simulink model "monosim"  (Simulink 7.7)
settings: Solver=ode45  StartTime=0.0  StopTime=10.0  MaxStep=0.01  RelTol=1e-3
values from neighbouring files (symbols this model uses):
  beta = 0.001    [teste.m]
undefined symbols (not defined in the file or in its folder): J, K, T
settings Model: Creator=ClaudiaPinto  LastModifiedBy=ClaudiaPinto

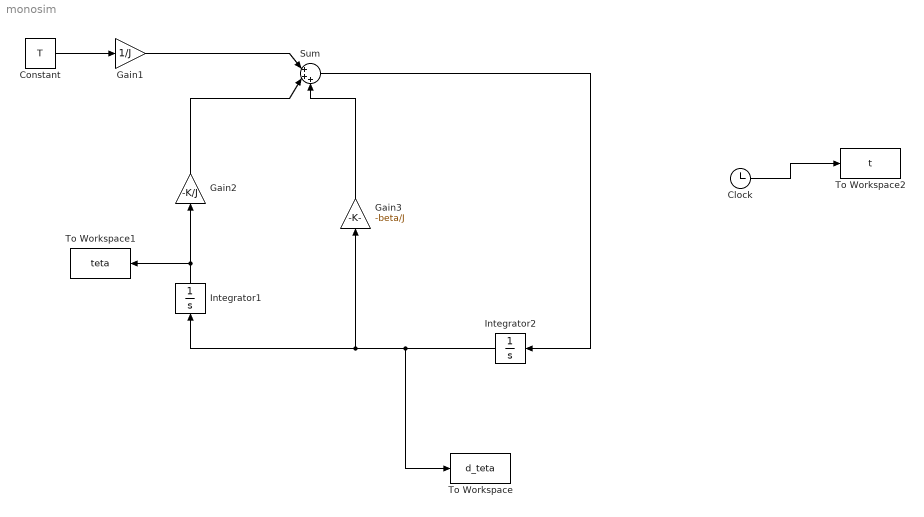
== system monosim ==
  Clock : Clock
      settings: Decimation=10
  Constant : Constant  Value=T
  Gain1 : Gain  Gain=1/J
  Gain2 : Gain  Gain=-K/J
  Gain3 : Gain  Gain=-beta/J
  Integrator1 : Integrator  InitialCondition=pi/4
  Integrator2 : Integrator
  Sum : Sum  Inputs=|+++
  To Workspace : ToWorkspace  VariableName=d_teta  SampleTime=-1  SaveFormat=Array
  To Workspace1 : ToWorkspace  VariableName=teta  SampleTime=-1  SaveFormat=Array
  To Workspace2 : ToWorkspace  VariableName=t  SampleTime=-1  SaveFormat=Array
  wires:
  Constant/1 -> Gain1/1
  Gain1/1 -> Sum/1
  Gain2/1 -> Sum/2
  Integrator1/1 -> Gain2/1, To Workspace1/1
  Integrator2/1 -> Integrator1/1, Gain3/1, To Workspace/1
  Gain3/1 -> Sum/3
  Sum/1 -> Integrator2/1
  Clock/1 -> To Workspace2/1
